simulink model "lab2_CL"  (R2016b)
settings: Solver=ode3  StartTime=0.0  StopTime=10.0  FixedStep=0.01  RelTol=1e-3  EnableMultiTasking=on
values from neighbouring files (symbols this model uses):
  kz3 = 1.73    [Lab2.m]
  z3 = z1 / 3    [Lab2.m]
libraries: arduinolib x4, neural x1
settings Model: ExtModeTrigDuration=2  Creator=MSI  LastModifiedBy=EE103
settings OptimizationCC: MaxStackSize=64
settings DebuggingCC: ParameterTunabilityLossMsg=error  SFExecutionAtInitializationDiag=none
settings HardwareCC: ProdBitPerInt=16  ProdBitPerPointer=16  ProdBitPerSizeT=16  ProdBitPerPtrDiffT=16  ProdLargestAtomicFloat=None  ProdWordSize=8  ProdHWDeviceType=Atmel->AVR
settings SFSimCC: SimUseLocalCustomCode=on
settings RTWCC: SystemTargetFile=ert.tlc  HardwareBoard=Arduino Uno  TLCOptions=-aInlineSetEventsForThisBaseRateFcn=TLC_FALSE -aSuppressMultiTaskScheduler=TLC_FALSE -aRateBasedStepFcn=1  TemplateMakefile=ert_default_tmf  Description=Embedded Coder  GenerateReport=on  RTWUseLocalCustomCode=on  Toolchain=Arduino AVR v1.6.7  BuildConfiguration=Faster Runs  IncludeHyperlinkInReport=on  LaunchReport=on  GenerateTraceInfo=on  GenerateTraceReport=on  GenerateTraceReportSl=on  GenerateTraceReportSf=on  GenerateTraceReportEml=on
settings CodeAppCC: ForceParamTrailComments=on  IgnoreCustomStorageClasses=off  OperatorAnnotations=on  SimulinkDataObjDesc=on  SFDataObjDesc=on  MATLABFcnDesc=on  InsertBlockDesc=on  MATLABSourceComments=on
settings ERTTargetCC: SupportContinuousTime=on  SupportVariableSizeSignals=on

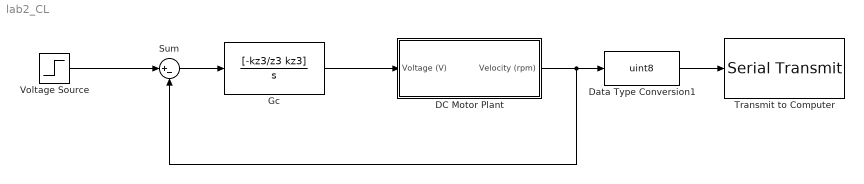
== system lab2_CL ==
  DC Motor Plant : Subsystem
  Data Type Conversion1 : DataTypeConversion  OutDataTypeStr=uint8  RndMeth=Round
  Gc : TransferFcn  Numerator=[-kz3/z3 kz3]  Denominator=[1 0]
  Sum : Sum  Inputs=|+-
  Transmit to Computer : arduinolib/Serial Transmit  portNumber=0  blockPlatform=arduino
  Voltage Source : Step  Time=0  After=50  SampleTime=0.01
  wires:
  Voltage Source/1 -> Sum/1
  Sum/1 -> Gc/1
  Gc/1 -> DC Motor Plant/1(Voltage (V))
  Data Type Conversion1/1 -> Transmit to Computer/1
  DC Motor Plant/1(Velocity (rpm)) -> Sum/2, Data Type Conversion1/1

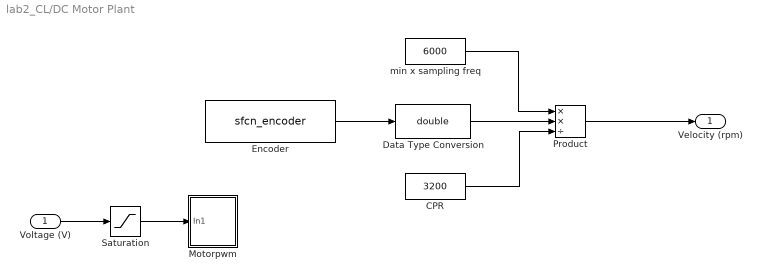
== system lab2_CL/DC Motor Plant ==
  Voltage (V) : Inport
  CPR : Constant  Value=3200
  Data Type Conversion : DataTypeConversion  OutDataTypeStr=double  RndMeth=Round
  Encoder : S-Function  InitFcn=try, set_param(gcb,'FunctionName','sfcn_encoder'), end  FunctionName=sfcn_encoder  Parameters=uint8(0),uint8(2),uint8(3)  SFunctionModules=sfcn_encoder_wrapper  SFunctionDeploymentMode=off  EnableBusSupport=off  mask(S-Function Builder){}
      mask init:
      | val = [[.9  0.75 0.75 1 1 .9 .9 1]',[1 1 0.75 0.75 .9 .9 1 .9]'];try , sys = get_param(gcb,'SfunBuilderFcnName');if isempty(sys), sys = get_param(gcb,'FunctionName'); end,catch, sys = get_param(gcb,'FunctionName'); end
      settings: CopyFcn=set_param(gcbh,'LinkStatus','none')  PreSaveFcn=try, set_param(gcb,'FunctionName','sfcn_encoder'), end  OpenFcn=sfunctionwizard(gcbh)
      mask Display: plot(val(:,1),val(:,2)),disp(sys), port_label('output',1,'pos')
  Motorpwm : Subsystem
  Product : Product  Inputs=**/
  Saturation : Saturate  UpperLimit=12  LowerLimit=-12
  min x sampling freq : Constant  Value=6000
  Velocity (rpm) : Outport
  wires:
  Encoder/1 -> Data Type Conversion/1
  Voltage (V)/1 -> Saturation/1
  Data Type Conversion/1 -> Product/2
  Product/1 -> Velocity (rpm)/1
  min x sampling freq/1 -> Product/1
  CPR/1 -> Product/3
  Saturation/1 -> Motorpwm/1(In1)

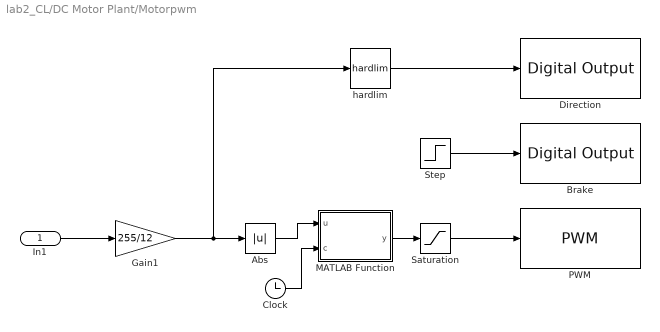
== system lab2_CL/DC Motor Plant/Motorpwm ==
  In1 : Inport
  Abs : Abs
  Brake : arduinolib/Digital Output  pinNumber=8  blockPlatform=arduino
  Clock : Clock
  "Direction " : arduinolib/Digital Output  pinNumber=13  blockPlatform=arduino
  Gain1 : Gain  Gain=255/12
  MATLAB Function : MATLAB Function  TreatAsAtomicUnit=on
  PWM : arduinolib/PWM  pinNumber=11  blockPlatform=arduino
  Saturation : Saturate  UpperLimit=255  LowerLimit=0
  Step : Step  Time=0  After=0  SampleTime=0
  hardlim : neural/Transfer Functions/hardlim
  wires:
  hardlim/1 -> "Direction "/1
  Step/1 -> Brake/1
  Saturation/1 -> PWM/1
  In1/1 -> Gain1/1
  MATLAB Function/1(y) -> Saturation/1
  Abs/1 -> MATLAB Function/1(u)
  Clock/1 -> MATLAB Function/2(c)
  Gain1/1 -> hardlim/1, Abs/1

== matlab function lab2_CL/DC Motor Plant/Motorpwm/MATLAB Function ==
  data: u input; y output; c input
function y = fcn(u,c)
%#codegen
if c<10
    y = u;
else
    y=0;
end
